simulink model "fsm"  (R2020a)
settings: Solver=FixedStepDiscrete  StartTime=0.0  StopTime=inf  FixedStep=Ts  MaxStep=0.01  RelTol=1e-3
model workspace (MAT data in the model file):
  Ts = 0.01
  blinking_period = 1
  debounce_tmo = 0.5
  test_tmo = 5
undefined symbols (not defined in the file or in its folder): StateButton
Description:
  | Ventilator Controller
settings Model: Creator=upattacini  LastModifiedBy=upattacini
settings SolverCC: MaxConsecutiveMinStep=10
settings DataIOCC: SaveOutput=off  SignalLogging=off  DSMLogging=off  SaveTime=off  ReturnWorkspaceOutputs=off
settings OptimizationCC: DefaultUnderspecifiedDataType=single  StrengthReduction=on  ZeroExternalMemoryAtStartup=off  ZeroInternalMemoryAtStartup=off  OptimizeBlockOrder=speed  OptimizationPriority=Speed  OptimizationCustomize=off  MultiThreadedLoops=on  EfficientTunableParamExpr=on
settings DebuggingCC: ParameterTunabilityLossMsg=error
settings SFSimCC: MATLABDynamicMemAlloc=off
settings RTWCC: SystemTargetFile=ert.tlc  GenCodeOnly=on  PackageGeneratedCodeAndArtifacts=on  PackageName=fsm  TemplateMakefile=ert_default_tmf  TargetLang=C++
settings CodeAppCC: ForceParamTrailComments=on  IgnoreCustomStorageClasses=off  OperatorAnnotations=on  SimulinkDataObjDesc=on  SFDataObjDesc=on  InsertBlockDesc=on
settings ERTTargetCC: TargetLangStandard=C++03 (ISO)  GenerateSampleERTMain=on  MultiInstanceERTCode=on  CodeInterfacePackaging=C++ class  RootIOFormat=Structure reference  ERTCustomFileTemplate=example_file_process.tlc

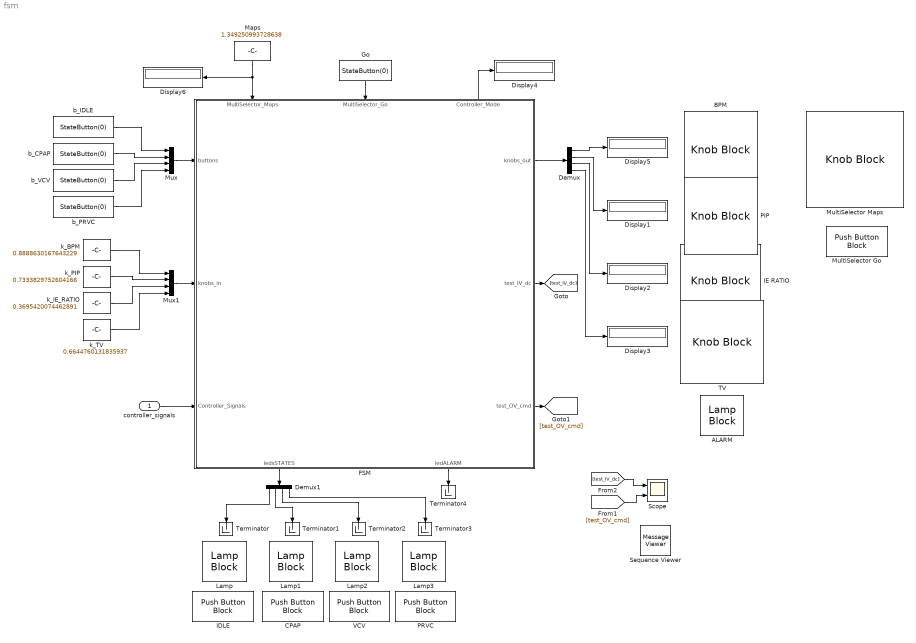
== system fsm ==
  controller_signals : Inport
  ALARM : LampBlock  LabelPosition=Hide
  BPM : KnobBlock  LabelPosition=Hide  ScaleMax=1
  CPAP : PushButtonBlock
  Demux : Demux
  Demux1 : Demux
  Display{1..6} (6 alike) : Display
  FSM : Subsystem  TreatAsAtomicUnit=on
      settings: PortSchema="{\"entries\":[{\"content\":{\"sides\":[{\"content\":{\"connectorIds\":[\"In1\",\"In2\",\"In3\"]},\"type\":\"ConnectorPlacement.EquallySpacedRectSide\",\"uuid\":\"c74e0fd1-2a09-4eed-97e5-23e0421db126\"},{\"content\":{\"connectorIds\":[\"Out1\",\"Out2\",\"Out3\"],\"side\":\"RIGHT\"},\"type\":\"ConnectorPlacement.EquallySpacedRectSide\",\"uuid\":\"36157922-0ce9-4b1e-9834-d3b675aa4f61\"},{\"content\":{\"connectorIds\":[\"In4\",\"In5\",\"Out6\"],\"side\":\"TOP\"},\"type\":\"ConnectorPlacement.EquallySpacedRectSide\",\"uuid\":\"35e50056-72b5-4d65-a91d-c8e9cd398685\"},{\"content\":{\"connectorIds\":[\"Out4\",\"Out5\"],\"side\":\"BOTTOM\"},\"type\":\"ConnectorPlacement.EquallySpacedRectSide\",\"uuid\":\"e3697b41-0a6c-42dd-91e3-5aa057d35a6e\"}]},\"type\":\"ConnectorPlacement.EquallySpacedConnector\",\"uuid\":\"1e2991a1-3462-4987-ab9d-18430a1f96c8\"}],\"packageUris\":[\"http://schema.mathworks.com/mf0/Connector/19700101\"],\"version\":\"1.0\"}"
  Go : Constant  Value=StateButton(0)  OutDataTypeStr=Enum: StateButton
  IDLE : PushButtonBlock
  IE RATIO : KnobBlock  LabelPosition=Hide  ScaleMax=1
  Lamp{,1..3} (4 alike) : LampBlock  LabelPosition=Hide
  Maps : Constant  Value=1.349250993728638  OutDataTypeStr=uint32
  MultiSelector Go : PushButtonBlock
  MultiSelector Maps : KnobBlock  LabelPosition=Hide  ScaleMin=1  ScaleMax=10  TickInterval=1
  Mux : Mux
  Mux1 : Mux
  PIP : KnobBlock  LabelPosition=Hide  ScaleMax=1
  PRVC : PushButtonBlock
  Scope : Scope  NumInputPorts=2
  Sequence Viewer : MessageViewer  VariableStepTimePrecision=5  History=10000
  TV : KnobBlock  LabelPosition=Hide  ScaleMax=1
  Terminator{,1..4} (5 alike) : Terminator
  VCV : PushButtonBlock
  b_CPAP : Constant  Value=StateButton(0)  OutDataTypeStr=Enum: StateButton
  b_IDLE : Constant  Value=StateButton(0)  OutDataTypeStr=Enum: StateButton
  b_PRVC : Constant  Value=StateButton(0)  OutDataTypeStr=Enum: StateButton
  b_VCV : Constant  Value=StateButton(0)  OutDataTypeStr=Enum: StateButton
  k_BPM : Constant  Value=0.8888630167643229  OutDataTypeStr=single
  k_IE_RATIO : Constant  Value=0.3695420074462891  OutDataTypeStr=single
  k_PIP : Constant  Value=0.7333829752604166  OutDataTypeStr=single
  k_TV : Constant  Value=0.6644760131835937  OutDataTypeStr=single
  wires:
  b_IDLE/1 -> Mux/1
  b_CPAP/1 -> Mux/2
  b_VCV/1 -> Mux/3
  b_PRVC/1 -> Mux/4
  k_PIP/1 -> Mux1/2
  k_IE_RATIO/1 -> Mux1/3
  k_BPM/1 -> Mux1/1
  k_TV/1 -> Mux1/4
  Demux/3 -> Display2/1
  Demux/2 -> Display1/1
  Demux/4 -> Display3/1
  Demux/1 -> Display5/1
  Demux1/1 -> Terminator/1
  Demux1/2 -> Terminator1/1
  Demux1/3 -> Terminator2/1
  Demux1/4 -> Terminator3/1
  [test_IV_dc] -> Scope/1
  [test_OV_cmd] -> Scope/2
  Mux/1 -> FSM/1(buttons)
  Mux1/1 -> FSM/2(knobs_in)
  controller_signals/1 -> FSM/3(Controller_Signals)
  Maps/1 -> Display6/1, FSM/4(MultiSelector_Maps)
  Go/1 -> FSM/5(MultiSelector_Go)
  FSM/6(Controller_Mode) -> Display4/1
  FSM/5(ledALARM) -> Terminator4/1
  FSM/4(ledsSTATES) -> Demux1/1
  FSM/3(test_OV_cmd) -> [test_OV_cmd]
  FSM/2(test_IV_dc) -> [test_IV_dc]
  FSM/1(knobs_out) -> Demux/1

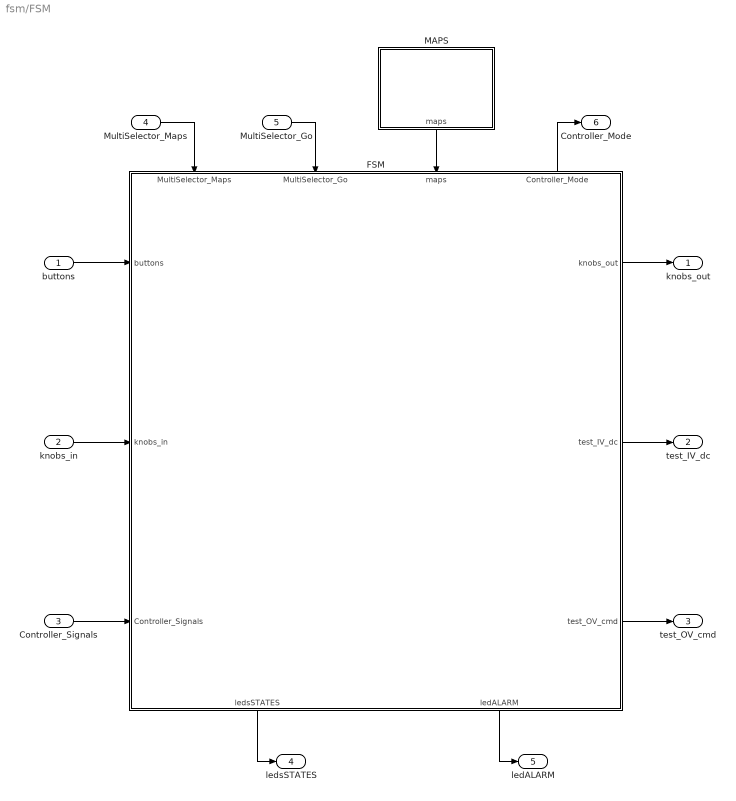
== system fsm/FSM ==
  buttons : Inport
  knobs_in : Inport  Port=2
  Controller_Signals : Inport  Port=3
  MultiSelector_Maps : Inport  Port=4
  MultiSelector_Go : Inport  Port=5
  FSM : Stateflow chart  TreatAsAtomicUnit=on
      settings: PortSchema="{\"entries\":[{\"content\":{\"sides\":[{\"content\":{\"connectorIds\":[\"In1\",\"In2\",\"In4\"]},\"type\":\"ConnectorPlacement.EquallySpacedRectSide\",\"uuid\":\"9fe4d650-a42b-4914-81a9-f70d7e6bcc0e\"},{\"content\":{\"connectorIds\":[\"Out2\",\"Out5\",\"Out6\"],\"side\":\"RIGHT\"},\"type\":\"ConnectorPlacement.EquallySpacedRectSide\",\"uuid\":\"3ee9ff79-e579-4e16-894f-9974c82009bd\"},{\"content\":{\"connectorIds\":[\"In3\",\"In5\",\"In6\",\"Out3\"],\"side\":\"TOP\"},\"type\":\"ConnectorPlacement.EquallySpacedRectSide\",\"uuid\":\"9d778e65-499e-4be9-a647-bfbc6362ac8b\"},{\"content\":{\"connectorIds\":[\"Out1\",\"Out4\"],\"side\":\"BOTTOM\"},\"type\":\"ConnectorPlacement.EquallySpacedRectSide\",\"uuid\":\"26e212ed-828c-4521-8cb5-d3de72989edb\"}]},\"type\":\"ConnectorPlacement.EquallySpacedConnector\",\"uuid\":\"b99c80d0-f016-4d09-b7d1-171101517ad5\"}],\"packageUris\":[\"http://schema.mathworks.com/mf0/Connector/19700101\"],\"version\":\"1.0\"}"
  MAPS : Subsystem
  knobs_out : Outport
  test_IV_dc : Outport  Port=2
  test_OV_cmd : Outport  Port=3
  ledsSTATES : Outport  Port=4
  ledALARM : Outport  Port=5
  Controller_Mode : Outport  Port=6
  wires:
  FSM/6(test_OV_cmd) -> test_OV_cmd/1
  FSM/3(Controller_Mode) -> Controller_Mode/1
  FSM/4(ledALARM) -> ledALARM/1
  Controller_Signals/1 -> FSM/4(Controller_Signals)
  buttons/1 -> FSM/1(buttons)
  knobs_in/1 -> FSM/2(knobs_in)
  FSM/5(test_IV_dc) -> test_IV_dc/1
  FSM/2(knobs_out) -> knobs_out/1
  FSM/1(ledsSTATES) -> ledsSTATES/1
  MultiSelector_Go/1 -> FSM/5(MultiSelector_Go)
  MultiSelector_Maps/1 -> FSM/3(MultiSelector_Maps)
  MAPS/1(maps) -> FSM/6(maps)

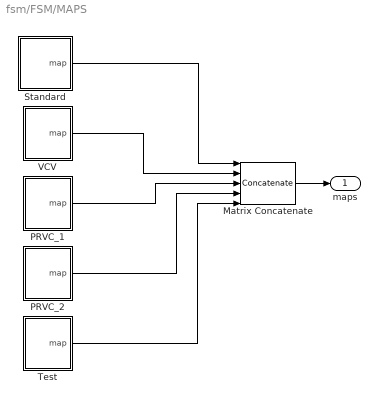
== system fsm/FSM/MAPS ==
  Matrix Concatenate : Concatenate  NumInputs=5  Mode=Multidimensional array  ConcatenateDimension=2
  PRVC_1 : Subsystem
  PRVC_2 : Subsystem
  Standard : Subsystem
  Test : Subsystem
  VCV : Subsystem
  maps : Outport
  wires:
  Standard/1(map) -> Matrix Concatenate/1
  VCV/1(map) -> Matrix Concatenate/2
  Matrix Concatenate/1 -> maps/1
  PRVC_1/1(map) -> Matrix Concatenate/3
  PRVC_2/1(map) -> Matrix Concatenate/4
  Test/1(map) -> Matrix Concatenate/5

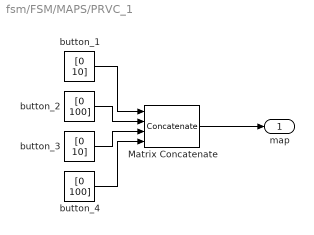
== system fsm/FSM/MAPS/PRVC_1 ==
  Matrix Concatenate : Concatenate  NumInputs=4  Mode=Multidimensional array  ConcatenateDimension=2
  button_1 : Constant  Value=[0 10]  OutDataTypeStr=single
  button_2 : Constant  Value=[0 100]  OutDataTypeStr=single
  button_3 : Constant  Value=[0 10]  OutDataTypeStr=single
  button_4 : Constant  Value=[0 100]  OutDataTypeStr=single
  map : Outport
  wires:
  Matrix Concatenate/1 -> map/1
  button_1/1 -> Matrix Concatenate/1
  button_4/1 -> Matrix Concatenate/4
  button_2/1 -> Matrix Concatenate/2
  button_3/1 -> Matrix Concatenate/3

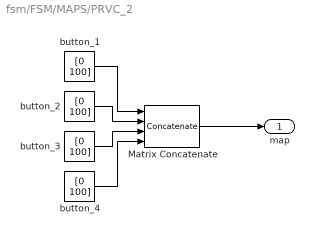
== system fsm/FSM/MAPS/PRVC_2 ==
  Matrix Concatenate : Concatenate  NumInputs=4  Mode=Multidimensional array  ConcatenateDimension=2
  button_{1..4} (4 alike) : Constant  Value=[0 100]  OutDataTypeStr=single
  map : Outport
  wires:
  button_3/1 -> Matrix Concatenate/3
  button_2/1 -> Matrix Concatenate/2
  button_4/1 -> Matrix Concatenate/4
  button_1/1 -> Matrix Concatenate/1
  Matrix Concatenate/1 -> map/1

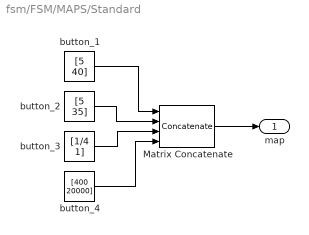
== system fsm/FSM/MAPS/Standard ==
  Matrix Concatenate : Concatenate  NumInputs=4  Mode=Multidimensional array  ConcatenateDimension=2
  button_1 : Constant  Value=[5 40]  OutDataTypeStr=single
  button_2 : Constant  Value=[5 35]  OutDataTypeStr=single
  button_3 : Constant  Value=[1/4 1]  OutDataTypeStr=single
  button_4 : Constant  Value=[400 20000]  OutDataTypeStr=single
  map : Outport
  wires:
  button_2/1 -> Matrix Concatenate/2
  button_3/1 -> Matrix Concatenate/3
  button_1/1 -> Matrix Concatenate/1
  button_4/1 -> Matrix Concatenate/4
  Matrix Concatenate/1 -> map/1

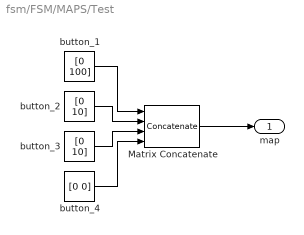
== system fsm/FSM/MAPS/Test ==
  Matrix Concatenate : Concatenate  NumInputs=4  Mode=Multidimensional array  ConcatenateDimension=2
  button_1 : Constant  Value=[0 100]  OutDataTypeStr=single
  button_2 : Constant  Value=[0 10]  OutDataTypeStr=single
  button_3 : Constant  Value=[0 10]  OutDataTypeStr=single
  button_4 : Constant  Value=[0 0]  OutDataTypeStr=single
  map : Outport
  wires:
  Matrix Concatenate/1 -> map/1
  button_1/1 -> Matrix Concatenate/1
  button_4/1 -> Matrix Concatenate/4
  button_2/1 -> Matrix Concatenate/2
  button_3/1 -> Matrix Concatenate/3

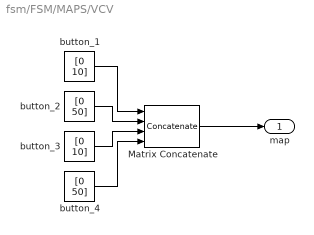
== system fsm/FSM/MAPS/VCV ==
  Matrix Concatenate : Concatenate  NumInputs=4  Mode=Multidimensional array  ConcatenateDimension=2
  button_1 : Constant  Value=[0 10]  OutDataTypeStr=single
  button_2 : Constant  Value=[0 50]  OutDataTypeStr=single
  button_3 : Constant  Value=[0 10]  OutDataTypeStr=single
  button_4 : Constant  Value=[0 50]  OutDataTypeStr=single
  map : Outport
  wires:
  button_3/1 -> Matrix Concatenate/3
  button_2/1 -> Matrix Concatenate/2
  button_4/1 -> Matrix Concatenate/4
  button_1/1 -> Matrix Concatenate/1
  Matrix Concatenate/1 -> map/1

== stateflow chart fsm/FSM/FSM ==
  state ALARMS_HANDLING [parallel]
    settings: executionOrder=2
    state INIT
      entry:
    (default) -> ALARMS_HANDLING.INIT
  state STATES_HANDLING [parallel]
    settings: executionOrder=1
    state TEST [group]
      state IDLE
        entry:
        ledsSTATES[ControlMode.CPAP] = StateLed.Off;
        ledsSTATES[ControlMode.VCV] = StateLed.Off;
        ledsSTATES[ControlMode.PRVC] = StateLed.Off;
        test_IV_dc = 0;
        test_OV_cmd = false;
        during:
        apply_map(MapIndex.MAP_Test);
        test1_dc_peak = knobs_out[0];
        test1_period = knobs_out[1];
        test2_period = knobs_out[2];
        ledsSTATES[ControlMode.PRVC] = unavailable_button(buttons[ControlMode.PRVC]);
      state TEST_1
        entry:
        test_IV_dc = 0;
        test_OV_cmd = true;
        ledsSTATES[ControlMode.CPAP] = StateLed.On;
        during:
        test_IV_dc += (test1_dc_peak / test1_period) * Ts;
        ledsSTATES[ControlMode.VCV] = unavailable_button(buttons[ControlMode.VCV]);
        ledsSTATES[ControlMode.PRVC] = unavailable_button(buttons[ControlMode.PRVC]);
      state TEST_2
        entry:
        test_IV_dc = 100;
        ledsSTATES[ControlMode.VCV] = StateLed.On;
        during:
        ledsSTATES[ControlMode.CPAP] = unavailable_button(buttons[ControlMode.CPAP]);
        ledsSTATES[ControlMode.PRVC] = unavailable_button(buttons[ControlMode.PRVC]);
      STATES_HANDLING.TEST.IDLE -> STATES_HANDLING.TEST.IDLE [order 4] : [!exit_test && (duration(buttons[ControlMode.IDLE]==StateButton.Released) >= debounce_tmo)]{exit_test=true;}
      STATES_HANDLING.TEST.IDLE -> TEST_1 [order 1] : [duration(buttons[ControlMode.CPAP]==StateButton.Pressed) >= debounce_tmo]
      TEST_1 -> STATES_HANDLING.TEST.IDLE [order 1] : [duration(buttons[ControlMode.IDLE]==StateButton.Pressed) >= debounce_tmo]{exit_test=false;}
      TEST_2 -> STATES_HANDLING.TEST.IDLE [order 1] : [duration(buttons[ControlMode.IDLE]==StateButton.Pressed) >= debounce_tmo]{exit_test=false;}
      STATES_HANDLING.TEST.IDLE -> TEST_2 [order 3] : [duration(buttons[ControlMode.VCV]==StateButton.Pressed) >= debounce_tmo]
      TEST_1 -> TEST_1 [order 2] : after(test1_period,sec)
      TEST_2 -> TEST_2 [order 2] : after(test2_period,sec)/test_OV_cmd = !test_OV_cmd;
    state INIT
      entry:
    state IDLE
      entry:
      ledsSTATES[ControlMode.IDLE] = StateLed.On;
      ledsSTATES[ControlMode.CPAP] = StateLed.Off;
      ledsSTATES[ControlMode.VCV] = StateLed.Off;
      ledsSTATES[ControlMode.PRVC] = StateLed.Off;
      Controller_Mode = ControlMode.IDLE;
      during:
      apply_map(MultiSelector_Maps_latch);
    state CPAP
      entry:
      ledsSTATES[ControlMode.IDLE] = StateLed.Off;
      ledsSTATES[ControlMode.CPAP] = StateLed.On;
      Controller_Mode = ControlMode.CPAP;
      during:
      ledsSTATES[ControlMode.VCV] = unavailable_button(buttons[ControlMode.VCV]);
      ledsSTATES[ControlMode.PRVC] = unavailable_button(buttons[ControlMode.PRVC]);
    state PRVC
      entry:
      ledsSTATES[ControlMode.IDLE] = StateLed.Off;
      ledsSTATES[ControlMode.PRVC] = StateLed.On;
      Controller_Mode = ControlMode.PRVC;
      during:
      ledsSTATES[ControlMode.CPAP] = unavailable_button(buttons[ControlMode.CPAP]);
      ledsSTATES[ControlMode.VCV] = unavailable_button(buttons[ControlMode.VCV]);
    state VCV
      entry:
      ledsSTATES[ControlMode.IDLE] = StateLed.Off;
      ledsSTATES[ControlMode.VCV] = StateLed.On;
      Controller_Mode = ControlMode.VCV;
      during:
      ledsSTATES[ControlMode.CPAP] = unavailable_button(buttons[ControlMode.CPAP]);
      ledsSTATES[ControlMode.PRVC] = unavailable_button(buttons[ControlMode.PRVC]);
    STATES_HANDLING.IDLE -> STATES_HANDLING.TEST.IDLE [order 4] : [enter_test && duration(buttons[ControlMode.IDLE]==StateButton.Pressed) >= test_tmo]{enter_test=false;}/send(blink_IDLE_on);
    (default) -> STATES_HANDLING.INIT
    STATES_HANDLING.TEST.IDLE -> STATES_HANDLING.IDLE [order 2] : [exit_test && duration(buttons[ControlMode.IDLE]==StateButton.Pressed) >= test_tmo]{exit_test=false;}/send(blink_IDLE_off);
    STATES_HANDLING.INIT -> STATES_HANDLING.IDLE
    STATES_HANDLING.IDLE -> STATES_HANDLING.IDLE [order 5] : [!enter_test && (duration(buttons[ControlMode.IDLE]==StateButton.Released) >= debounce_tmo)]{enter_test=true;}
    CPAP -> STATES_HANDLING.IDLE [order 1] : idle_controller
    STATES_HANDLING.IDLE -> CPAP [order 1] : [duration(buttons[ControlMode.CPAP]==StateButton.Pressed) >= debounce_tmo]{enter_test=false;}
    VCV -> STATES_HANDLING.IDLE [order 2] : [duration(buttons[ControlMode.IDLE]==StateButton.Pressed) >= debounce_tmo]{enter_test=false;}
    CPAP -> STATES_HANDLING.IDLE [order 2] : [duration(buttons[ControlMode.IDLE]==StateButton.Pressed) >= debounce_tmo]
    STATES_HANDLING.IDLE -> VCV [order 2] : [duration(buttons[ControlMode.VCV]==StateButton.Pressed) >= debounce_tmo]
    VCV -> STATES_HANDLING.IDLE [order 1] : idle_controller
    STATES_HANDLING.IDLE -> STATES_HANDLING.IDLE [order 6] : [duration(MultiSelector_Go==StateButton.Pressed) >= debounce_tmo]{latch_multiselector();}
    STATES_HANDLING.IDLE -> PRVC [order 3] : [duration(buttons[ControlMode.PRVC]==StateButton.Pressed) >= debounce_tmo]
    PRVC -> STATES_HANDLING.IDLE [order 1] : idle_controller
    PRVC -> STATES_HANDLING.IDLE [order 2] : [duration(buttons[ControlMode.IDLE]==StateButton.Pressed) >= debounce_tmo]{enter_test=false;}
  state IDLE_BLINKING [parallel]
    settings: executionOrder=3
    state INIT
      entry:
      ledsSTATES[ControlMode.IDLE] = StateLed.Off;
    state ON
      entry:
      ledsSTATES[ControlMode.IDLE] = StateLed.On;
    state OFF
      entry:
      ledsSTATES[ControlMode.IDLE] = StateLed.Off;
    (default) -> IDLE_BLINKING.INIT
    IDLE_BLINKING.INIT -> ON : blink_IDLE_on
    OFF -> IDLE_BLINKING.INIT [order 2] : blink_IDLE_off
    ON -> IDLE_BLINKING.INIT [order 2] : blink_IDLE_off
    OFF -> ON [order 1] : after(blinking_period,sec)
    ON -> OFF [order 1] : after(blinking_period,sec)
  data: n function_input double; test1_dc_peak local single size=1; test1_period local single size=1; test2_period local single size=1; debounce_tmo parameter single size=1; test_tmo parameter single size=1; enter_test local boolean =false; exit_test local boolean =false; state function_input double; led function_output double; buttons input Enum: StateButton size=4; ledsSTATES output Enum: StateLed size=4; knobs_in input single size=4 [0..1]; MultiSelector_Maps input uint32 size=1 [1..10]; knobs_out output single size=4; Controller_Mode output Enum: ControlMode size=1; ledALARM output Enum: StateLed; test_IV_dc output single; test_OV_cmd output boolean; blinking_period parameter single size=1; Ts parameter single; Controller_Signals input single size=9; MultiSelector_Go input Enum: StateButton size=1 [0..100]; maps input single size=[2 20]; map_min local single size=4; map_max local single size=4; MultiSelector_Maps_latch local uint32 size=1 =1
  data Controller_Signals settings: description=|
      | Signals order:
      | - S1_P
      | - S2_Q
      | - S3_P
      | - S3_T
      | - S4_P
      | - S5_Q
      | - S7_P
      | - V_lungs_measured
      | - trigger
      | 
      | Units:
      | - P = [cmH2O]
      | - Q = [L/min]
      | - V = [L]
  events: blink_IDLE_on local FUNCTION_CALL_EVENT; blink_IDLE_off local FUNCTION_CALL_EVENT; idle_controller local FUNCTION_CALL_EVENT
  function apply_map(n):
    | function apply_map(n)
    | 
    | for i = 1:4
    |     j = 4*(n-1)+i;
    |     knobs_out(i) = maps(1, j) + knobs_in(i) * (maps(2, j) - maps(1, j));
    | end
  function latch_multiselector:
    | function latch_multiselector()
    | 
    | if MultiSelector_Maps < 1
    |     MultiSelector_Maps_latch = uint32(1);
    | elseif MultiSelector_Maps > length(maps)
    |     MultiSelector_Maps_latch = uint32(length(maps));
    | else
    |     MultiSelector_Maps_latch = MultiSelector_Maps;
    | end
  function led = unavailable_button(state):
    | function led = unavailable_button(state)
    | 
    | if state == StateButton.Pressed
    |     led = double(StateLed.On);
    | else
    |     led = double(StateLed.Off);
    | end
